simulink library "ddm"  (R2021b)
settings: Solver=VariableStepAuto  StartTime=0.0  StopTime=10.0  RelTol=1e-3
undefined symbols (not defined in the file or in its folder): ADDM_FrTMTqDev_X_Nm, ADDM_RrTMTqDev_X_Nm, ENUM_ADASACCSTA_ERROR, ENUM_ADASACCSTA_OFF, ENUM_ADASACCSTA_STANDBY, ENUM_ALLOWMOV_ALLOWREADY, ENUM_APS, ENUM_BRKSTA_ERROR, ENUM_BRKSTA_OFF, ENUM_BRKSTA_ON, ENUM_BRKSW_INVALID, ENUM_BRKSW_OFF, ENUM_BRKSW_ON, ENUM_CHGPREACTERRSTA_OBCPRE, ENUM_DCDCFAULTSTA_ANYFAULTLV1, ENUM_DCDCFAULTSTA_ANYFAULTLV2, ENUM_DRIVETRAIN_AWD, ENUM_DRIVETRAIN_FWD, ENUM_DRIVETRAIN_RWD, ENUM_EDUDRTSTA_NORMAL, ENUM_EPBSTA_APPLIED, ENUM_EPBSTA_RELEASED, ENUM_GEARACTUALPOSN_INVALID, ENUM_GEARACTUALPOSN_P, ENUM_HVBATTREADYPRE_READY, ENUM_MCUWARN_LV0, ENUM_MCUWARN_LV1, ENUM_MCUWARN_LV2, ENUM_MCUWARN_LV3, ENUM_MCUWARN_NOERROR, ENUM_OBCFAULTSTA_ANYFAULT, ENUM_PAS_R2F2, ENUM_PDFAULT_BATTPDFAIL, ENUM_PDFAULT_DCDCDISABLE, ENUM_PDFAULT_MCUDISABLE, ENUM_PDFAULT_MCUDISCHRG, ENUM_POWERSTA_OFF, ENUM_POWERSTA_ON, ENUM_POWERSTA_READY, ENUM_POWERSTA_STANDBY, ENUM_PRESSINDI_LOW, ENUM_PUFAULT_BATTUPFAIL, ENUM_PUFAULT_DCDCENABLEFAIL, ENUM_PUFAULT_PRECHRGCHKFAIL, ENUM_PUFAULT_SAFETYCHKFAIL, ENUM_PUSTATE_COMPLETED, ENUM_PWRSTASW_OFF, ENUM_PWRSTASW_OFFA, ENUM_PWRSTASW_OFFCHVCHRG, ENUM_PWRSTASW_OFFCLVCHRG, ENUM_PWRSTASW_ON, ENUM_PWRSTASW_ONHVCHRG, ENUM_PWRSTASW_READY, ENUM_PWRSTASW_STANDBY, ENUM_SHIFTCOMMAND_P, ENUM_SHIFTERERRSTA_PBUTTONFAILURE, ENUM_VEHMALFUNLV_2ND, ENUM_VEHMALFUNLV_3RD, ENUM_VEHMALFUNLV_4TH, ENUM_VEHMALFUNLV_NORMAL ... (+459)
libraries: hcu_lib x515, simulink x3
(part 10 of 25)

== system ddm/DDM/DDM/TPM/LFWheelTmpHigh ==
  note: Test Detection Criteria
  note: Test Pass Criteria
  note: Release Condition After Decision
  note: Diagnostics and Fault Handling
  task_time_s : Inport
  VPMM_PowerSta_enum : Inport  Port=2
  DTC_clear_request : Inport  Port=3
  VTPM_LFWheelTmpHigh_flg : Inport  Port=4
  Constant : Constant  Value=KDDM_LFWheelTmpHighDTC_cnt
  Constant1 : Constant  Value=KDDM_LFWheelTmpHighDTC_cnt
  Constant10 : Constant  Value=ENUM_POWERSTA_OFF
  Constant11 : Constant  Value=KDDM_LFWheelTmpHighPassSW_flg
  Constant12 : Constant  Value=FALSE
  Constant13 : Constant  Value=KDDM_LFWheelTmpHighCFSSW_flg
  Constant14 : Constant  Value=KDDM_LFWheelTmpHighDFSSW_flg
  Constant15 : Constant  Value=KDDM_LFWheelTmpHighPassTO_s
  Constant2 : Constant  Value=ENUM_POWERSTA_READY
  Constant24 : Constant  Value=TRUE
  Constant25 : Constant  Value=FALSE
  Constant3 : Constant  Value=ENUM_POWERSTA_ON
  Constant4 : Constant  Value=FALSE
  Constant46 : Constant  Value=KDDM_LFWheelTmpHighDetSW_flg
  Constant5 : Constant  Value=ENUM_POWERSTA_READY
  Constant6 : Constant  Value=KDDM_LFWheelTmpHighDetTO_s
  Constant7 : Constant  Value=ENUM_POWERSTA_ON
  Constant8 : Constant  Value=TRUE
  Constant9 : Constant  Value=KDDM_LFWheelTmpHighPassTO_s
  DTC_Couter : hcu_lib/Basic_Blocks/DTC_Couter
  DTC_Info : hcu_lib/Basic_Blocks/DTC_Info
  Data Type Conversion1 : DataTypeConversion  OutDataTypeStr=uint8
  Equal{1..5} (5 alike) : RelationalOperator  Operator===  OutDataTypeStr=boolean  RndMeth=Simplest
  Equal6 : RelationalOperator  OutDataTypeStr=boolean  RndMeth=Simplest
  Logical Operator{1,4..5,7..8} (5 alike) : Logic  Operator=OR  AllPortsSameDT=off  OutDataTypeStr=boolean
  Logical Operator12 : Logic  AllPortsSameDT=off  OutDataTypeStr=boolean
  Logical Operator15 : Logic  AllPortsSameDT=off  OutDataTypeStr=boolean
  Logical Operator18 : Logic  AllPortsSameDT=off  OutDataTypeStr=boolean
  Logical Operator19 : Logic  Inputs=3  AllPortsSameDT=off  OutDataTypeStr=boolean
  Logical Operator2 : Logic  Operator=NOT  AllPortsSameDT=off  OutDataTypeStr=boolean
  Logical Operator3 : Logic  Operator=OR  Inputs=3  AllPortsSameDT=off  OutDataTypeStr=boolean
  Logical Operator6 : Logic  Operator=NOT  AllPortsSameDT=off  OutDataTypeStr=boolean
  Relay : Relay  OnSwitchValue=ONE_INT  OffSwitchValue=ZERO_INT
  SR_Latch1 : Subsystem  mask(SR_Latch){}
      mask help: SR latch function.
  SR_Latch3 : hcu_lib/Basic_Blocks/SR_Latch
  SR_Latch4 : hcu_lib/Basic_Blocks/SR_Latch
  Switch{2..4,6} (4 alike) : Switch  Criteria=u2 ~= 0
  Test Detection Criteria : hcu_lib/Basic_Blocks/Test Detection Criteria
  Timer1 : hcu_lib/Basic_Blocks/Timer
  VDDM_LFWheelTmpHighDTC_raw32 : Outport
  wires:
  [VTPM_LFWheelTmpHigh_flg] -> Switch4/1
  [VTPM_LFWheelTmpHigh_flg] -> Switch3/1
  task_time_s/1 -> [task_time_s]
  VPMM_PowerSta_enum/1 -> [VPMM_PowerSta_enum]
  Logical Operator8/1 -> Switch2/2
  Constant25/1 -> Switch2/3
  Switch2/1 -> [VDDM_LFWheelTmpHighCFSRls_flg]
  [DTC_clear_request] -> Logical Operator8/2
  Constant24/1 -> Switch2/1
  Constant10/1 -> Equal4/2
  Equal4/1 -> Logical Operator8/1
  [VDDM_LFWheelTmpHighDTC_cnt] -> Relay/1
  [VDDM_LFWheelTmpHighCFS_flg] -> Logical Operator7/1
  Logical Operator3/1 -> Logical Operator15/1
  [VDDM_LFWheelTmpHighDet_flg] -> Logical Operator19/1
  Relay/1 -> SR_Latch3/1
  DTC_Couter/2 -> Data Type Conversion1/1
  Constant1/1 -> DTC_Couter/3
  Logical Operator15/1 -> DTC_Couter/2
  Constant11/1 -> Logical Operator15/2
  Logical Operator19/1 -> DTC_Couter/1
  Constant46/1 -> Logical Operator19/2
  Data Type Conversion1/1 -> [VDDM_LFWheelTmpHighDTC_cnt]  "VDDM_LFWheelTmpHighDTC_cnt"
  DTC_Couter/1 -> SR_Latch4/1
  [VDDM_LFWheelTmpHighPass_flg] -> Logical Operator3/2
  [VDDM_LFWheelTmpHighCFSRls_flg] -> Logical Operator5/1
  SR_Latch4/1 -> Logical Operator18/1
  Logical Operator12/1 -> [VDDM_LFWheelTmpHighDFS_flg]
  Constant13/1 -> Logical Operator18/2
  SR_Latch3/1 -> Logical Operator12/2
  Constant14/1 -> Logical Operator12/1
  Logical Operator18/1 -> [VDDM_LFWheelTmpHighCFS_flg]
  [VDDM_LFWheelTmpHighCFSRls_flg] -> Logical Operator3/3
  DTC_clear_request/1 -> [DTC_clear_request]
  [VPMM_PowerSta_enum] -> Equal4/1
  [VDDM_LFWheelTmpHighCFS_flg] -> DTC_Info/3
  DTC_Info/1 -> VDDM_LFWheelTmpHighDTC_raw32/1  "VDDM_LFWheelTmpHighDTC_raw32"
  Test Detection Criteria/1 -> [VDDM_LFWheelTmpHighDet_flg]  "VDDM_LFWheelTmpHighDet_flg"
  [VDDM_LFWheelTmpHighDet_flg] -> DTC_Info/1
  [VDDM_LFWheelTmpHighPass_flg] -> DTC_Info/2
  [DTC_clear_request] -> DTC_Info/4
  [VPMM_PowerSta_enum] -> Equal1/1
  Constant4/1 -> Switch3/3
  Constant5/1 -> Equal1/2
  Constant7/1 -> Equal5/2
  Logical Operator1/1 -> Switch3/2
  Equal5/1 -> Logical Operator1/1
  Equal1/1 -> Logical Operator1/2
  [VPMM_PowerSta_enum] -> Equal5/1
  Constant6/1 -> Test Detection Criteria/4
  Constant/1 -> Test Detection Criteria/3
  [task_time_s] -> Test Detection Criteria/2
  [VPMM_PowerSta_enum] -> Equal3/1
  Equal2/1 -> Logical Operator4/2
  Constant8/1 -> Switch4/3
  Constant2/1 -> Equal2/2
  Constant3/1 -> Equal3/2
  [VPMM_PowerSta_enum] -> Equal2/1
  Equal3/1 -> Logical Operator4/1
  Logical Operator4/1 -> Switch4/2
  VTPM_LFWheelTmpHigh_flg/1 -> [VTPM_LFWheelTmpHigh_flg]
  Switch3/1 -> [VDDM_LFWheelTmpHighChk_flg], Switch6/3
  [DTC_clear_request] -> Switch6/2
  Constant12/1 -> Switch6/1
  Switch6/1 -> Test Detection Criteria/1
  Switch4/1 -> Timer1/2, Logical Operator6/1
  Equal6/1 -> SR_Latch1/1(set)
  Constant9/1 -> Equal6/2
  SR_Latch1/1(latched) -> [VDDM_LFWheelTmpHighPass_flg]
  [VDDM_LFWheelTmpHighChk_flg] -> SR_Latch1/2(reset)
  [task_time_s] -> Timer1/3
  Timer1/1 -> Equal6/1
  Constant15/1 -> Timer1/4
  Logical Operator6/1 -> Timer1/1
  Logical Operator2/1 -> Logical Operator19/3
  [DTC_clear_request] -> Logical Operator3/1, Logical Operator2/1
  Logical Operator5/1 -> SR_Latch4/2
  [DTC_clear_request] -> Logical Operator5/2
  Logical Operator7/1 -> SR_Latch3/2
  [DTC_clear_request] -> Logical Operator7/2

== system ddm/DDM/DDM/TPM/LRBatwarn ==
  note: Test Detection Criteria
  note: Test Pass Criteria
  note: Release Condition After Decision
  note: Diagnostics and Fault Handling
  task_time_s : Inport
  VPMM_PowerSta_enum : Inport  Port=2
  DTC_clear_request : Inport  Port=3
  VTPM_LRBatwarn_flg : Inport  Port=4
  Constant : Constant  Value=KDDM_LRBatwarnDTC_cnt
  Constant1 : Constant  Value=KDDM_LRBatwarnDTC_cnt
  Constant10 : Constant  Value=ENUM_POWERSTA_OFF
  Constant11 : Constant  Value=KDDM_LRBatwarnPassSW_flg
  Constant12 : Constant  Value=FALSE
  Constant13 : Constant  Value=KDDM_LRBatwarnCFSSW_flg
  Constant14 : Constant  Value=KDDM_LRBatwarnDFSSW_flg
  Constant15 : Constant  Value=KDDM_LRBatwarnPassTO_s
  Constant2 : Constant  Value=ENUM_POWERSTA_READY
  Constant24 : Constant  Value=TRUE
  Constant25 : Constant  Value=FALSE
  Constant3 : Constant  Value=ENUM_POWERSTA_ON
  Constant4 : Constant  Value=FALSE
  Constant46 : Constant  Value=KDDM_LRBatwarnDetSW_flg
  Constant5 : Constant  Value=ENUM_POWERSTA_READY
  Constant6 : Constant  Value=KDDM_LRBatwarnDetTO_s
  Constant7 : Constant  Value=ENUM_POWERSTA_ON
  Constant8 : Constant  Value=TRUE
  Constant9 : Constant  Value=KDDM_LRBatwarnPassTO_s
  DTC_Couter : hcu_lib/Basic_Blocks/DTC_Couter
  DTC_Info : hcu_lib/Basic_Blocks/DTC_Info
  Data Type Conversion1 : DataTypeConversion  OutDataTypeStr=uint8
  Equal{1..5} (5 alike) : RelationalOperator  Operator===  OutDataTypeStr=boolean  RndMeth=Simplest
  Equal6 : RelationalOperator  OutDataTypeStr=boolean  RndMeth=Simplest
  Logical Operator{1..2,4,7..8} (5 alike) : Logic  Operator=OR  AllPortsSameDT=off  OutDataTypeStr=boolean
  Logical Operator12 : Logic  AllPortsSameDT=off  OutDataTypeStr=boolean
  Logical Operator15 : Logic  AllPortsSameDT=off  OutDataTypeStr=boolean
  Logical Operator18 : Logic  AllPortsSameDT=off  OutDataTypeStr=boolean
  Logical Operator19 : Logic  Inputs=3  AllPortsSameDT=off  OutDataTypeStr=boolean
  Logical Operator3 : Logic  Operator=OR  Inputs=3  AllPortsSameDT=off  OutDataTypeStr=boolean
  Logical Operator5 : Logic  Operator=NOT  AllPortsSameDT=off  OutDataTypeStr=boolean
  Logical Operator6 : Logic  Operator=NOT  AllPortsSameDT=off  OutDataTypeStr=boolean
  Relay : Relay  OnSwitchValue=ONE_INT  OffSwitchValue=ZERO_INT
  SR_Latch1 : Subsystem  mask(SR_Latch){}
      mask help: SR latch function.
  SR_Latch3 : hcu_lib/Basic_Blocks/SR_Latch
  SR_Latch4 : hcu_lib/Basic_Blocks/SR_Latch
  Switch{2..4,6} (4 alike) : Switch  Criteria=u2 ~= 0
  Test Detection Criteria : hcu_lib/Basic_Blocks/Test Detection Criteria
  Timer1 : hcu_lib/Basic_Blocks/Timer
  VDDM_LRBatwarnDTC_raw32 : Outport
  wires:
  task_time_s/1 -> [task_time_s]
  VPMM_PowerSta_enum/1 -> [VPMM_PowerSta_enum]
  Logical Operator8/1 -> Switch2/2
  Constant25/1 -> Switch2/3
  Switch2/1 -> [VDDM_LRBatwarnCFSRls_flg]
  [DTC_clear_request] -> Logical Operator8/2
  Constant24/1 -> Switch2/1
  Constant10/1 -> Equal4/2
  Equal4/1 -> Logical Operator8/1
  [VDDM_LRBatwarnDTC_cnt] -> Relay/1
  [VDDM_LRBatwarnCFS_flg] -> Logical Operator7/1
  Logical Operator3/1 -> Logical Operator15/1
  [VDDM_LRBatwarnDet_flg] -> Logical Operator19/1
  Relay/1 -> SR_Latch3/1
  DTC_Couter/2 -> Data Type Conversion1/1
  Constant1/1 -> DTC_Couter/3
  Logical Operator15/1 -> DTC_Couter/2
  Constant11/1 -> Logical Operator15/2
  Logical Operator19/1 -> DTC_Couter/1
  Constant46/1 -> Logical Operator19/2
  Data Type Conversion1/1 -> [VDDM_LRBatwarnDTC_cnt]  "VDDM_LRBatwarnDTC_cnt"
  DTC_Couter/1 -> SR_Latch4/1
  [VDDM_LRBatwarnPass_flg] -> Logical Operator3/2
  [VDDM_LRBatwarnCFSRls_flg] -> Logical Operator2/1
  SR_Latch4/1 -> Logical Operator18/1
  Logical Operator12/1 -> [VDDM_LRBatwarnDFS_flg]
  Constant13/1 -> Logical Operator18/2
  SR_Latch3/1 -> Logical Operator12/2
  Constant14/1 -> Logical Operator12/1
  Logical Operator18/1 -> [VDDM_LRBatwarnCFS_flg]
  [VDDM_LRBatwarnCFSRls_flg] -> Logical Operator3/3
  DTC_clear_request/1 -> [DTC_clear_request]
  [VPMM_PowerSta_enum] -> Equal4/1
  [VDDM_LRBatwarnCFS_flg] -> DTC_Info/3
  DTC_Info/1 -> VDDM_LRBatwarnDTC_raw32/1  "VDDM_LRBatwarnDTC_raw32"
  Test Detection Criteria/1 -> [VDDM_LRBatwarnDet_flg]  "VDDM_LRBatwarnDet_flg"
  [VDDM_LRBatwarnDet_flg] -> DTC_Info/1
  [VDDM_LRBatwarnPass_flg] -> DTC_Info/2
  [DTC_clear_request] -> DTC_Info/4
  [VPMM_PowerSta_enum] -> Equal1/1
  Constant4/1 -> Switch3/3
  Constant2/1 -> Equal1/2
  Constant3/1 -> Equal5/2
  Logical Operator1/1 -> Switch3/2
  Equal5/1 -> Logical Operator1/1
  Equal1/1 -> Logical Operator1/2
  [VPMM_PowerSta_enum] -> Equal5/1
  Constant6/1 -> Test Detection Criteria/4
  Constant/1 -> Test Detection Criteria/3
  [task_time_s] -> Test Detection Criteria/2
  [VTPM_LRBatwarn_flg] -> Switch3/1
  [VPMM_PowerSta_enum] -> Equal3/1
  Equal2/1 -> Logical Operator4/2
  Constant8/1 -> Switch4/3
  Constant5/1 -> Equal2/2
  Constant7/1 -> Equal3/2
  [VPMM_PowerSta_enum] -> Equal2/1
  Equal3/1 -> Logical Operator4/1
  Logical Operator4/1 -> Switch4/2
  [VTPM_LRBatwarn_flg] -> Switch4/1
  VTPM_LRBatwarn_flg/1 -> [VTPM_LRBatwarn_flg]
  [DTC_clear_request] -> Switch6/2
  Constant12/1 -> Switch6/1
  Switch6/1 -> Test Detection Criteria/1
  Switch4/1 -> Timer1/2, Logical Operator6/1
  Equal6/1 -> SR_Latch1/1(set)
  [VDDM_LRBatwarnChk_flg] -> SR_Latch1/2(reset)
  Timer1/1 -> Equal6/1
  Constant9/1 -> Equal6/2
  SR_Latch1/1(latched) -> [VDDM_LRBatwarnPass_flg]
  [task_time_s] -> Timer1/3
  Logical Operator6/1 -> Timer1/1
  Constant15/1 -> Timer1/4
  Switch3/1 -> [VDDM_LRBatwarnChk_flg], Switch6/3
  Logical Operator5/1 -> Logical Operator19/3
  [DTC_clear_request] -> Logical Operator3/1, Logical Operator5/1
  Logical Operator2/1 -> SR_Latch4/2
  [DTC_clear_request] -> Logical Operator2/2
  Logical Operator7/1 -> SR_Latch3/2
  [DTC_clear_request] -> Logical Operator7/2

== system ddm/DDM/DDM/TPM/LRPressureLow ==
  note: Diagnostics and Fault Handling
  note: Release Condition After Decision
  note: Test Pass Criteria
  note: Test Detection Criteria
  task_time_s : Inport
  VPMM_PowerSta_enum : Inport  Port=2
  DTC_clear_request : Inport  Port=3
  VTPM_LRPressIndi_enum : Inport  Port=4
  Constant : Constant  Value=KDDM_LRPressIndiDTC_cnt
  Constant1 : Constant  Value=KDDM_LRPressIndiDTC_cnt
  Constant10 : Constant  Value=ENUM_POWERSTA_OFF
  Constant11 : Constant  Value=KDDM_LRPressIndiPassSW_flg
  Constant12 : Constant  Value=FALSE
  Constant13 : Constant  Value=KDDM_LRPressIndiCFSSW_flg
  Constant14 : Constant  Value=KDDM_LRPressIndiDFSSW_flg
  Constant15 : Constant  Value=KDDM_LRPressIndiPassTO_s
  Constant16 : Constant  Value=ENUM_PRESSINDI_LOW
  Constant17 : Constant  Value=ENUM_PRESSINDI_LOW
  Constant2 : Constant  Value=ENUM_POWERSTA_READY
  Constant24 : Constant  Value=TRUE
  Constant25 : Constant  Value=FALSE
  Constant3 : Constant  Value=ENUM_POWERSTA_ON
  Constant4 : Constant  Value=FALSE
  Constant46 : Constant  Value=KDDM_LRPressIndiDetSW_flg
  Constant5 : Constant  Value=ENUM_POWERSTA_READY
  Constant6 : Constant  Value=KDDM_LRPressIndiDetTO_s
  Constant7 : Constant  Value=ENUM_POWERSTA_ON
  Constant8 : Constant  Value=TRUE
  Constant9 : Constant  Value=KDDM_LRPressIndiPassTO_s
  DTC_Couter : hcu_lib/Basic_Blocks/DTC_Couter
  DTC_Info : hcu_lib/Basic_Blocks/DTC_Info
  Data Type Conversion1 : DataTypeConversion  OutDataTypeStr=uint8
  Equal{1..5,7..8} (7 alike) : RelationalOperator  Operator===  OutDataTypeStr=boolean  RndMeth=Simplest
  Equal6 : RelationalOperator  OutDataTypeStr=boolean  RndMeth=Simplest
  Logical Operator{1,4..5,7..8} (5 alike) : Logic  Operator=OR  AllPortsSameDT=off  OutDataTypeStr=boolean
  Logical Operator12 : Logic  AllPortsSameDT=off  OutDataTypeStr=boolean
  Logical Operator15 : Logic  AllPortsSameDT=off  OutDataTypeStr=boolean
  Logical Operator18 : Logic  AllPortsSameDT=off  OutDataTypeStr=boolean
  Logical Operator19 : Logic  Inputs=3  AllPortsSameDT=off  OutDataTypeStr=boolean
  Logical Operator2 : Logic  Operator=NOT  AllPortsSameDT=off  OutDataTypeStr=boolean
  Logical Operator3 : Logic  Operator=OR  Inputs=3  AllPortsSameDT=off  OutDataTypeStr=boolean
  Logical Operator6 : Logic  Operator=NOT  AllPortsSameDT=off  OutDataTypeStr=boolean
  Relay : Relay  OnSwitchValue=ONE_INT  OffSwitchValue=ZERO_INT
  SR_Latch1 : Subsystem  mask(SR_Latch){}
      mask help: SR latch function.
  SR_Latch3 : hcu_lib/Basic_Blocks/SR_Latch
  SR_Latch4 : hcu_lib/Basic_Blocks/SR_Latch
  Switch{2..4,6} (4 alike) : Switch  Criteria=u2 ~= 0
  Test Detection Criteria : hcu_lib/Basic_Blocks/Test Detection Criteria
  Timer1 : hcu_lib/Basic_Blocks/Timer
  VDDM_LRPressIndiDTC_raw32 : Outport
  wires:
  Logical Operator6/1 -> Timer1/1
  Constant15/1 -> Timer1/4
  Timer1/1 -> Equal6/1
  [task_time_s] -> Timer1/3
  [VDDM_LRPressIndiChk_flg] -> SR_Latch1/2(reset)
  SR_Latch1/1(latched) -> [VDDM_LRPressIndiPass_flg]
  Constant9/1 -> Equal6/2
  Equal6/1 -> SR_Latch1/1(set)
  Switch4/1 -> Timer1/2, Logical Operator6/1
  Switch6/1 -> Test Detection Criteria/1
  Constant12/1 -> Switch6/1
  [DTC_clear_request] -> Switch6/2
  Switch3/1 -> Switch6/3, [VDDM_LRPressIndiChk_flg]
  VTPM_LRPressIndi_enum/1 -> [VTPM_LRPressIndi_enum]
  Logical Operator4/1 -> Switch4/2
  Equal3/1 -> Logical Operator4/1
  [VPMM_PowerSta_enum] -> Equal2/1
  Constant3/1 -> Equal3/2
  Constant2/1 -> Equal2/2
  Constant8/1 -> Switch4/3
  Equal2/1 -> Logical Operator4/2
  [VPMM_PowerSta_enum] -> Equal3/1
  [task_time_s] -> Test Detection Criteria/2
  Constant/1 -> Test Detection Criteria/3
  Constant6/1 -> Test Detection Criteria/4
  [VPMM_PowerSta_enum] -> Equal5/1
  Equal1/1 -> Logical Operator1/2
  Equal5/1 -> Logical Operator1/1
  Logical Operator1/1 -> Switch3/2
  Constant7/1 -> Equal5/2
  Constant5/1 -> Equal1/2
  Constant4/1 -> Switch3/3
  [VPMM_PowerSta_enum] -> Equal1/1
  [DTC_clear_request] -> DTC_Info/4
  [VDDM_LRPressIndiPass_flg] -> DTC_Info/2
  [VDDM_LRPressIndiDet_flg] -> DTC_Info/1
  Test Detection Criteria/1 -> [VDDM_LRPressIndiDet_flg]  "VDDM_LRPressIndiDet_flg"
  DTC_Info/1 -> VDDM_LRPressIndiDTC_raw32/1  "VDDM_LRPressIndiDTC_raw32"
  [VDDM_LRPressIndiCFS_flg] -> DTC_Info/3
  [VPMM_PowerSta_enum] -> Equal4/1
  DTC_clear_request/1 -> [DTC_clear_request]
  [VDDM_LRPressIndiCFSRls_flg] -> Logical Operator3/3
  Logical Operator18/1 -> [VDDM_LRPressIndiCFS_flg]
  Constant14/1 -> Logical Operator12/1
  SR_Latch3/1 -> Logical Operator12/2
  Constant13/1 -> Logical Operator18/2
  Logical Operator12/1 -> [VDDM_LRPressIndiDFS_flg]
  SR_Latch4/1 -> Logical Operator18/1
  [VDDM_LRPressIndiCFSRls_flg] -> Logical Operator5/1
  [VDDM_LRPressIndiPass_flg] -> Logical Operator3/2
  DTC_Couter/1 -> SR_Latch4/1
  Data Type Conversion1/1 -> [VDDM_LRPressIndiDTC_cnt]  "VDDM_LRPressIndiDTC_cnt"
  Constant46/1 -> Logical Operator19/2
  Logical Operator19/1 -> DTC_Couter/1
  Constant11/1 -> Logical Operator15/2
  Logical Operator15/1 -> DTC_Couter/2
  Constant1/1 -> DTC_Couter/3
  DTC_Couter/2 -> Data Type Conversion1/1
  Relay/1 -> SR_Latch3/1
  [VDDM_LRPressIndiDet_flg] -> Logical Operator19/1
  Logical Operator3/1 -> Logical Operator15/1
  [VDDM_LRPressIndiCFS_flg] -> Logical Operator7/1
  [VDDM_LRPressIndiDTC_cnt] -> Relay/1
  Equal4/1 -> Logical Operator8/1
  Constant10/1 -> Equal4/2
  Constant24/1 -> Switch2/1
  [DTC_clear_request] -> Logical Operator8/2
  Switch2/1 -> [VDDM_LRPressIndiCFSRls_flg]
  Constant25/1 -> Switch2/3
  Logical Operator8/1 -> Switch2/2
  VPMM_PowerSta_enum/1 -> [VPMM_PowerSta_enum]
  task_time_s/1 -> [task_time_s]
  [VTPM_LRPressIndi_enum] -> Equal7/1
  Equal7/1 -> Switch3/1
  Constant16/1 -> Equal7/2
  Equal8/1 -> Switch4/1
  Constant17/1 -> Equal8/2
  [VTPM_LRPressIndi_enum] -> Equal8/1
  Logical Operator2/1 -> Logical Operator19/3
  [DTC_clear_request] -> Logical Operator3/1, Logical Operator2/1
  Logical Operator5/1 -> SR_Latch4/2
  [DTC_clear_request] -> Logical Operator5/2
  Logical Operator7/1 -> SR_Latch3/2
  [DTC_clear_request] -> Logical Operator7/2

== system ddm/DDM/DDM/TPM/LRSensorfail ==
  note: Diagnostics and Fault Handling
  note: Release Condition After Decision
  note: Test Pass Criteria
  note: Test Detection Criteria
  task_time_s : Inport
  VPMM_PowerSta_enum : Inport  Port=2
  DTC_clear_request : Inport  Port=3
  VTPM_LRSensorFail_flg : Inport  Port=4
  Constant : Constant  Value=KDDM_LRSensorFailDTC_cnt
  Constant1 : Constant  Value=KDDM_LRSensorFailDTC_cnt
  Constant10 : Constant  Value=ENUM_POWERSTA_OFF
  Constant11 : Constant  Value=KDDM_LRSensorFailPassSW_flg
  Constant12 : Constant  Value=FALSE
  Constant13 : Constant  Value=KDDM_LRSensorFailCFSSW_flg
  Constant14 : Constant  Value=KDDM_LRSensorFailDFSSW_flg
  Constant15 : Constant  Value=KDDM_LRSensorFailPassTO_s
  Constant2 : Constant  Value=ENUM_POWERSTA_READY
  Constant24 : Constant  Value=TRUE
  Constant25 : Constant  Value=FALSE
  Constant3 : Constant  Value=ENUM_POWERSTA_ON
  Constant4 : Constant  Value=FALSE
  Constant46 : Constant  Value=KDDM_LRSensorFailDetSW_flg
  Constant5 : Constant  Value=ENUM_POWERSTA_READY
  Constant6 : Constant  Value=KDDM_LRSensorFailDetTO_s
  Constant7 : Constant  Value=ENUM_POWERSTA_ON
  Constant8 : Constant  Value=TRUE
  Constant9 : Constant  Value=KDDM_LRSensorFailPassTO_s
  DTC_Couter : hcu_lib/Basic_Blocks/DTC_Couter
  DTC_Info : hcu_lib/Basic_Blocks/DTC_Info
  Data Type Conversion1 : DataTypeConversion  OutDataTypeStr=uint8
  Equal{1..5} (5 alike) : RelationalOperator  Operator===  OutDataTypeStr=boolean  RndMeth=Simplest
  Equal6 : RelationalOperator  OutDataTypeStr=boolean  RndMeth=Simplest
  Logical Operator{1,4..5,7..8} (5 alike) : Logic  Operator=OR  AllPortsSameDT=off  OutDataTypeStr=boolean
  Logical Operator12 : Logic  AllPortsSameDT=off  OutDataTypeStr=boolean
  Logical Operator15 : Logic  AllPortsSameDT=off  OutDataTypeStr=boolean
  Logical Operator18 : Logic  AllPortsSameDT=off  OutDataTypeStr=boolean
  Logical Operator19 : Logic  Inputs=3  AllPortsSameDT=off  OutDataTypeStr=boolean
  Logical Operator2 : Logic  Operator=NOT  AllPortsSameDT=off  OutDataTypeStr=boolean
  Logical Operator3 : Logic  Operator=OR  Inputs=3  AllPortsSameDT=off  OutDataTypeStr=boolean
  Logical Operator6 : Logic  Operator=NOT  AllPortsSameDT=off  OutDataTypeStr=boolean
  Relay : Relay  OnSwitchValue=ONE_INT  OffSwitchValue=ZERO_INT
  SR_Latch1 : Subsystem  mask(SR_Latch){}
      mask help: SR latch function.
  SR_Latch3 : hcu_lib/Basic_Blocks/SR_Latch
  SR_Latch4 : hcu_lib/Basic_Blocks/SR_Latch
  Switch{2..4,6} (4 alike) : Switch  Criteria=u2 ~= 0
  Test Detection Criteria : hcu_lib/Basic_Blocks/Test Detection Criteria
  Timer1 : hcu_lib/Basic_Blocks/Timer
  VDDM_LRSensorFailDTC_raw32 : Outport
  wires:
  Logical Operator6/1 -> Timer1/1
  Constant15/1 -> Timer1/4
  Timer1/1 -> Equal6/1
  [task_time_s] -> Timer1/3
  [VDDM_LRSensorFailChk_flg] -> SR_Latch1/2(reset)
  SR_Latch1/1(latched) -> [VDDM_LRSensorFailPass_flg]
  Constant9/1 -> Equal6/2
  Equal6/1 -> SR_Latch1/1(set)
  Switch4/1 -> Logical Operator6/1, Timer1/2
  Switch6/1 -> Test Detection Criteria/1
  Constant12/1 -> Switch6/1
  [DTC_clear_request] -> Switch6/2
  Switch3/1 -> Switch6/3, [VDDM_LRSensorFailChk_flg]
  VTPM_LRSensorFail_flg/1 -> [VTPM_LRSensorFail_flg]
  Logical Operator4/1 -> Switch4/2
  Equal3/1 -> Logical Operator4/1
  [VPMM_PowerSta_enum] -> Equal2/1
  Constant3/1 -> Equal3/2
  Constant2/1 -> Equal2/2
  Constant8/1 -> Switch4/3
  Equal2/1 -> Logical Operator4/2
  [VPMM_PowerSta_enum] -> Equal3/1
  [task_time_s] -> Test Detection Criteria/2
  Constant/1 -> Test Detection Criteria/3
  Constant6/1 -> Test Detection Criteria/4
  [VPMM_PowerSta_enum] -> Equal5/1
  Equal1/1 -> Logical Operator1/2
  Equal5/1 -> Logical Operator1/1
  Logical Operator1/1 -> Switch3/2
  Constant7/1 -> Equal5/2
  Constant5/1 -> Equal1/2
  Constant4/1 -> Switch3/3
  [VPMM_PowerSta_enum] -> Equal1/1
  [DTC_clear_request] -> DTC_Info/4
  [VDDM_LRSensorFailPass_flg] -> DTC_Info/2
  [VDDM_LRSensorFailDet_flg] -> DTC_Info/1
  Test Detection Criteria/1 -> [VDDM_LRSensorFailDet_flg]  "VDDM_LRSensorFailDet_flg"
  DTC_Info/1 -> VDDM_LRSensorFailDTC_raw32/1  "VDDM_LRSensorFailDTC_raw32"
  [VDDM_LRSensorFailCFS_flg] -> DTC_Info/3
  [VPMM_PowerSta_enum] -> Equal4/1
  DTC_clear_request/1 -> [DTC_clear_request]
  [VDDM_LRSensorFailCFSRls_flg] -> Logical Operator3/3
  Logical Operator18/1 -> [VDDM_LRSensorFailCFS_flg]
  Constant14/1 -> Logical Operator12/1
  SR_Latch3/1 -> Logical Operator12/2
  Constant13/1 -> Logical Operator18/2
  Logical Operator12/1 -> [VDDM_LRSensorFailDFS_flg]
  SR_Latch4/1 -> Logical Operator18/1
  [VDDM_LRSensorFailCFSRls_flg] -> Logical Operator5/1
  [VDDM_LRSensorFailPass_flg] -> Logical Operator3/2
  DTC_Couter/1 -> SR_Latch4/1
  Data Type Conversion1/1 -> [VDDM_LRSensorFailDTC_cnt]  "VDDM_LRSensorFailDTC_cnt"
  Constant46/1 -> Logical Operator19/2
  Logical Operator19/1 -> DTC_Couter/1
  Constant11/1 -> Logical Operator15/2
  Logical Operator15/1 -> DTC_Couter/2
  Constant1/1 -> DTC_Couter/3
  DTC_Couter/2 -> Data Type Conversion1/1
  Relay/1 -> SR_Latch3/1
  [VDDM_LRSensorFailDet_flg] -> Logical Operator19/1
  Logical Operator3/1 -> Logical Operator15/1
  [VDDM_LRSensorFailCFS_flg] -> Logical Operator7/1
  [VDDM_LRSensorFailDTC_cnt] -> Relay/1
  Equal4/1 -> Logical Operator8/1
  Constant10/1 -> Equal4/2
  Constant24/1 -> Switch2/1
  [DTC_clear_request] -> Logical Operator8/2
  Switch2/1 -> [VDDM_LRSensorFailCFSRls_flg]
  Constant25/1 -> Switch2/3
  Logical Operator8/1 -> Switch2/2
  VPMM_PowerSta_enum/1 -> [VPMM_PowerSta_enum]
  task_time_s/1 -> [task_time_s]
  [VTPM_LRSensorFail_flg] -> Switch3/1
  [VTPM_LRSensorFail_flg] -> Switch4/1
  Logical Operator2/1 -> Logical Operator19/3
  [DTC_clear_request] -> Logical Operator3/1, Logical Operator2/1
  Logical Operator5/1 -> SR_Latch4/2
  [DTC_clear_request] -> Logical Operator5/2
  Logical Operator7/1 -> SR_Latch3/2
  [DTC_clear_request] -> Logical Operator7/2

== system ddm/DDM/DDM/TPM/LRWheelTmpHigh ==
  note: Test Detection Criteria
  note: Test Pass Criteria
  note: Release Condition After Decision
  note: Diagnostics and Fault Handling
  task_time_s : Inport
  VPMM_PowerSta_enum : Inport  Port=2
  DTC_clear_request : Inport  Port=3
  VTPM_LRWheelTmpHigh_flg : Inport  Port=4
  Constant : Constant  Value=KDDM_LRWheelTmpHighDTC_cnt
  Constant1 : Constant  Value=KDDM_LRWheelTmpHighDTC_cnt
  Constant10 : Constant  Value=ENUM_POWERSTA_OFF
  Constant11 : Constant  Value=KDDM_LRWheelTmpHighPassSW_flg
  Constant12 : Constant  Value=FALSE
  Constant13 : Constant  Value=KDDM_LRWheelTmpHighCFSSW_flg
  Constant14 : Constant  Value=KDDM_LRWheelTmpHighDFSSW_flg
  Constant15 : Constant  Value=KDDM_LRWheelTmpHighPassTO_s
  Constant2 : Constant  Value=ENUM_POWERSTA_READY
  Constant24 : Constant  Value=TRUE
  Constant25 : Constant  Value=FALSE
  Constant3 : Constant  Value=ENUM_POWERSTA_ON
  Constant4 : Constant  Value=FALSE
  Constant46 : Constant  Value=KDDM_LRWheelTmpHighDetSW_flg
  Constant5 : Constant  Value=ENUM_POWERSTA_READY
  Constant6 : Constant  Value=KDDM_LRWheelTmpHighDetTO_s
  Constant7 : Constant  Value=ENUM_POWERSTA_ON
  Constant8 : Constant  Value=TRUE
  Constant9 : Constant  Value=KDDM_LRWheelTmpHighPassTO_s
  DTC_Couter : hcu_lib/Basic_Blocks/DTC_Couter
  DTC_Info : hcu_lib/Basic_Blocks/DTC_Info
  Data Type Conversion1 : DataTypeConversion  OutDataTypeStr=uint8
  Equal{1..5} (5 alike) : RelationalOperator  Operator===  OutDataTypeStr=boolean  RndMeth=Simplest
  Equal6 : RelationalOperator  OutDataTypeStr=boolean  RndMeth=Simplest
  Logical Operator{1,4..5,7..8} (5 alike) : Logic  Operator=OR  AllPortsSameDT=off  OutDataTypeStr=boolean
  Logical Operator12 : Logic  AllPortsSameDT=off  OutDataTypeStr=boolean
  Logical Operator15 : Logic  AllPortsSameDT=off  OutDataTypeStr=boolean
  Logical Operator18 : Logic  AllPortsSameDT=off  OutDataTypeStr=boolean
  Logical Operator19 : Logic  Inputs=3  AllPortsSameDT=off  OutDataTypeStr=boolean
  Logical Operator2 : Logic  Operator=NOT  AllPortsSameDT=off  OutDataTypeStr=boolean
  Logical Operator3 : Logic  Operator=OR  Inputs=3  AllPortsSameDT=off  OutDataTypeStr=boolean
  Logical Operator6 : Logic  Operator=NOT  AllPortsSameDT=off  OutDataTypeStr=boolean
  Relay : Relay  OnSwitchValue=ONE_INT  OffSwitchValue=ZERO_INT
  SR_Latch1 : Subsystem  mask(SR_Latch){}
      mask help: SR latch function.
  SR_Latch3 : hcu_lib/Basic_Blocks/SR_Latch
  SR_Latch4 : hcu_lib/Basic_Blocks/SR_Latch
  Switch{2..4,6} (4 alike) : Switch  Criteria=u2 ~= 0
  Test Detection Criteria : hcu_lib/Basic_Blocks/Test Detection Criteria
  Timer1 : hcu_lib/Basic_Blocks/Timer
  VDDM_LRWheelTmpHighDTC_raw32 : Outport
  wires:
  [VTPM_LRWheelTmpHigh_flg] -> Switch4/1
  [VTPM_LRWheelTmpHigh_flg] -> Switch3/1
  task_time_s/1 -> [task_time_s]
  VPMM_PowerSta_enum/1 -> [VPMM_PowerSta_enum]
  Logical Operator8/1 -> Switch2/2
  Constant25/1 -> Switch2/3
  Switch2/1 -> [VDDM_LRWheelTmpHighCFSRls_flg]
  [DTC_clear_request] -> Logical Operator8/2
  Constant24/1 -> Switch2/1
  Constant10/1 -> Equal4/2
  Equal4/1 -> Logical Operator8/1
  [VDDM_LRWheelTmpHighDTC_cnt] -> Relay/1
  [VDDM_LRWheelTmpHighCFS_flg] -> Logical Operator7/1
  Logical Operator3/1 -> Logical Operator15/1
  [VDDM_LRWheelTmpHighDet_flg] -> Logical Operator19/1
  Relay/1 -> SR_Latch3/1
  DTC_Couter/2 -> Data Type Conversion1/1
  Constant1/1 -> DTC_Couter/3
  Logical Operator15/1 -> DTC_Couter/2
  Constant11/1 -> Logical Operator15/2
  Logical Operator19/1 -> DTC_Couter/1
  Constant46/1 -> Logical Operator19/2
  Data Type Conversion1/1 -> [VDDM_LRWheelTmpHighDTC_cnt]  "VDDM_LRWheelTmpHighDTC_cnt"
  DTC_Couter/1 -> SR_Latch4/1
  [VDDM_LRWheelTmpHighPass_flg] -> Logical Operator3/2
  [VDDM_LRWheelTmpHighCFSRls_flg] -> Logical Operator5/1
  SR_Latch4/1 -> Logical Operator18/1
  Logical Operator12/1 -> [VDDM_LRWheelTmpHighDFS_flg]
  Constant13/1 -> Logical Operator18/2
  SR_Latch3/1 -> Logical Operator12/2
  Constant14/1 -> Logical Operator12/1
  Logical Operator18/1 -> [VDDM_LRWheelTmpHighCFS_flg]
  [VDDM_LRWheelTmpHighCFSRls_flg] -> Logical Operator3/3
  DTC_clear_request/1 -> [DTC_clear_request]
  [VPMM_PowerSta_enum] -> Equal4/1
  [VDDM_LRWheelTmpHighCFS_flg] -> DTC_Info/3
  DTC_Info/1 -> VDDM_LRWheelTmpHighDTC_raw32/1  "VDDM_LRWheelTmpHighDTC_raw32"
  Test Detection Criteria/1 -> [VDDM_LRWheelTmpHighDet_flg]  "VDDM_LRWheelTmpHighDet_flg"
  [VDDM_LRWheelTmpHighDet_flg] -> DTC_Info/1
  [VDDM_LRWheelTmpHighPass_flg] -> DTC_Info/2
  [DTC_clear_request] -> DTC_Info/4
  [VPMM_PowerSta_enum] -> Equal1/1
  Constant4/1 -> Switch3/3
  Constant5/1 -> Equal1/2
  Constant7/1 -> Equal5/2
  Logical Operator1/1 -> Switch3/2
  Equal5/1 -> Logical Operator1/1
  Equal1/1 -> Logical Operator1/2
  [VPMM_PowerSta_enum] -> Equal5/1
  Constant6/1 -> Test Detection Criteria/4
  Constant/1 -> Test Detection Criteria/3
  [task_time_s] -> Test Detection Criteria/2
  [VPMM_PowerSta_enum] -> Equal3/1
  Equal2/1 -> Logical Operator4/2
  Constant8/1 -> Switch4/3
  Constant2/1 -> Equal2/2
  Constant3/1 -> Equal3/2
  [VPMM_PowerSta_enum] -> Equal2/1
  Equal3/1 -> Logical Operator4/1
  Logical Operator4/1 -> Switch4/2
  VTPM_LRWheelTmpHigh_flg/1 -> [VTPM_LRWheelTmpHigh_flg]
  Switch3/1 -> [VDDM_LRWheelTmpHighChk_flg], Switch6/3
  [DTC_clear_request] -> Switch6/2
  Constant12/1 -> Switch6/1
  Switch6/1 -> Test Detection Criteria/1
  Switch4/1 -> Timer1/2, Logical Operator6/1
  Equal6/1 -> SR_Latch1/1(set)
  Constant9/1 -> Equal6/2
  SR_Latch1/1(latched) -> [VDDM_LRWheelTmpHighPass_flg]
  [VDDM_LRWheelTmpHighChk_flg] -> SR_Latch1/2(reset)
  [task_time_s] -> Timer1/3
  Timer1/1 -> Equal6/1
  Constant15/1 -> Timer1/4
  Logical Operator6/1 -> Timer1/1
  Logical Operator2/1 -> Logical Operator19/3
  [DTC_clear_request] -> Logical Operator3/1, Logical Operator2/1
  [DTC_clear_request] -> Logical Operator5/2
  Logical Operator5/1 -> SR_Latch4/2
  Logical Operator7/1 -> SR_Latch3/2
  [DTC_clear_request] -> Logical Operator7/2

== system ddm/DDM/DDM/TPM/RFBatwarn ==
  note: Diagnostics and Fault Handling
  note: Release Condition After Decision
  note: Test Pass Criteria
  note: Test Detection Criteria
  task_time_s : Inport
  VPMM_PowerSta_enum : Inport  Port=2
  DTC_clear_request : Inport  Port=3
  VTPM_RFBatwarn_flg : Inport  Port=4
  Constant : Constant  Value=KDDM_RFBatwarnDTC_cnt
  Constant1 : Constant  Value=KDDM_RFBatwarnDTC_cnt
  Constant10 : Constant  Value=ENUM_POWERSTA_OFF
  Constant11 : Constant  Value=KDDM_RFBatwarnPassSW_flg
  Constant12 : Constant  Value=FALSE
  Constant13 : Constant  Value=KDDM_RFBatwarnCFSSW_flg
  Constant14 : Constant  Value=KDDM_RFBatwarnDFSSW_flg
  Constant15 : Constant  Value=KDDM_RFBatwarnPassTO_s
  Constant2 : Constant  Value=ENUM_POWERSTA_READY
  Constant24 : Constant  Value=TRUE
  Constant25 : Constant  Value=FALSE
  Constant3 : Constant  Value=ENUM_POWERSTA_ON
  Constant4 : Constant  Value=FALSE
  Constant46 : Constant  Value=KDDM_RFBatwarnDetSW_flg
  Constant5 : Constant  Value=ENUM_POWERSTA_READY
  Constant6 : Constant  Value=KDDM_RFBatwarnDetTO_s
  Constant7 : Constant  Value=ENUM_POWERSTA_ON
  Constant8 : Constant  Value=TRUE
  Constant9 : Constant  Value=KDDM_RFBatwarnPassTO_s
  DTC_Couter : hcu_lib/Basic_Blocks/DTC_Couter
  DTC_Info : hcu_lib/Basic_Blocks/DTC_Info
  Data Type Conversion1 : DataTypeConversion  OutDataTypeStr=uint8
  Equal{1..5} (5 alike) : RelationalOperator  Operator===  OutDataTypeStr=boolean  RndMeth=Simplest
  Equal6 : RelationalOperator  OutDataTypeStr=boolean  RndMeth=Simplest
  Logical Operator{1,4..5,7..8} (5 alike) : Logic  Operator=OR  AllPortsSameDT=off  OutDataTypeStr=boolean
  Logical Operator12 : Logic  AllPortsSameDT=off  OutDataTypeStr=boolean
  Logical Operator15 : Logic  AllPortsSameDT=off  OutDataTypeStr=boolean
  Logical Operator18 : Logic  AllPortsSameDT=off  OutDataTypeStr=boolean
  Logical Operator19 : Logic  Inputs=3  AllPortsSameDT=off  OutDataTypeStr=boolean
  Logical Operator2 : Logic  Operator=NOT  AllPortsSameDT=off  OutDataTypeStr=boolean
  Logical Operator3 : Logic  Operator=OR  Inputs=3  AllPortsSameDT=off  OutDataTypeStr=boolean
  Logical Operator6 : Logic  Operator=NOT  AllPortsSameDT=off  OutDataTypeStr=boolean
  Relay : Relay  OnSwitchValue=ONE_INT  OffSwitchValue=ZERO_INT
  SR_Latch1 : Subsystem  mask(SR_Latch){}
      mask help: SR latch function.
  SR_Latch3 : hcu_lib/Basic_Blocks/SR_Latch
  SR_Latch4 : hcu_lib/Basic_Blocks/SR_Latch
  Switch{2..4,6} (4 alike) : Switch  Criteria=u2 ~= 0
  Test Detection Criteria : hcu_lib/Basic_Blocks/Test Detection Criteria
  Timer1 : hcu_lib/Basic_Blocks/Timer
  VDDM_RFBatwarnDTC_raw32 : Outport
  wires:
  Switch6/1 -> Test Detection Criteria/1
  Constant12/1 -> Switch6/1
  [DTC_clear_request] -> Switch6/2
  Switch3/1 -> [VDDM_RFBatwarnChk_flg], Switch6/3
  VTPM_RFBatwarn_flg/1 -> [VTPM_RFBatwarn_flg]
  [VTPM_RFBatwarn_flg] -> Switch4/1
  Logical Operator4/1 -> Switch4/2
  Equal3/1 -> Logical Operator4/1
  [VPMM_PowerSta_enum] -> Equal2/1
  Constant3/1 -> Equal3/2
  Constant2/1 -> Equal2/2
  Constant8/1 -> Switch4/3
  Equal2/1 -> Logical Operator4/2
  [VPMM_PowerSta_enum] -> Equal3/1
  [VTPM_RFBatwarn_flg] -> Switch3/1
  [task_time_s] -> Test Detection Criteria/2
  Constant/1 -> Test Detection Criteria/3
  Constant6/1 -> Test Detection Criteria/4
  [VPMM_PowerSta_enum] -> Equal5/1
  Equal1/1 -> Logical Operator1/2
  Equal5/1 -> Logical Operator1/1
  Logical Operator1/1 -> Switch3/2
  Constant7/1 -> Equal5/2
  Constant5/1 -> Equal1/2
  Constant4/1 -> Switch3/3
  [VPMM_PowerSta_enum] -> Equal1/1
  [DTC_clear_request] -> DTC_Info/4
  [VDDM_RFBatwarnPass_flg] -> DTC_Info/2
  [VDDM_RFBatwarnDet_flg] -> DTC_Info/1
  Test Detection Criteria/1 -> [VDDM_RFBatwarnDet_flg]  "VDDM_RFBatwarnDet_flg"
  DTC_Info/1 -> VDDM_RFBatwarnDTC_raw32/1  "VDDM_RFBatwarnDTC_raw32"
  [VDDM_RFBatwarnCFS_flg] -> DTC_Info/3
  [VPMM_PowerSta_enum] -> Equal4/1
  DTC_clear_request/1 -> [DTC_clear_request]
  [VDDM_RFBatwarnCFSRls_flg] -> Logical Operator3/3
  Logical Operator18/1 -> [VDDM_RFBatwarnCFS_flg]
  Constant14/1 -> Logical Operator12/1
  SR_Latch3/1 -> Logical Operator12/2
  Constant13/1 -> Logical Operator18/2
  Logical Operator12/1 -> [VDDM_RFBatwarnDFS_flg]
  SR_Latch4/1 -> Logical Operator18/1
  [VDDM_RFBatwarnCFSRls_flg] -> Logical Operator5/1
  [VDDM_RFBatwarnPass_flg] -> Logical Operator3/2
  DTC_Couter/1 -> SR_Latch4/1
  Data Type Conversion1/1 -> [VDDM_RFBatwarnDTC_cnt]  "VDDM_RFBatwarnDTC_cnt"
  Constant46/1 -> Logical Operator19/2
  Logical Operator19/1 -> DTC_Couter/1
  Constant11/1 -> Logical Operator15/2
  Logical Operator15/1 -> DTC_Couter/2
  Constant1/1 -> DTC_Couter/3
  DTC_Couter/2 -> Data Type Conversion1/1
  Relay/1 -> SR_Latch3/1
  [VDDM_RFBatwarnDet_flg] -> Logical Operator19/1
  Logical Operator3/1 -> Logical Operator15/1
  [VDDM_RFBatwarnCFS_flg] -> Logical Operator7/1
  [VDDM_RFBatwarnDTC_cnt] -> Relay/1
  Equal4/1 -> Logical Operator8/1
  Constant10/1 -> Equal4/2
  Constant24/1 -> Switch2/1
  [DTC_clear_request] -> Logical Operator8/2
  Switch2/1 -> [VDDM_RFBatwarnCFSRls_flg]
  Constant25/1 -> Switch2/3
  Logical Operator8/1 -> Switch2/2
  VPMM_PowerSta_enum/1 -> [VPMM_PowerSta_enum]
  task_time_s/1 -> [task_time_s]
  Switch4/1 -> Timer1/2, Logical Operator6/1
  Equal6/1 -> SR_Latch1/1(set)
  [VDDM_RFBatwarnChk_flg] -> SR_Latch1/2(reset)
  Timer1/1 -> Equal6/1
  Constant9/1 -> Equal6/2
  SR_Latch1/1(latched) -> [VDDM_RFBatwarnPass_flg]
  [task_time_s] -> Timer1/3
  Logical Operator6/1 -> Timer1/1
  Constant15/1 -> Timer1/4
  Logical Operator2/1 -> Logical Operator19/3
  [DTC_clear_request] -> Logical Operator3/1, Logical Operator2/1
  Logical Operator5/1 -> SR_Latch4/2
  [DTC_clear_request] -> Logical Operator5/2
  Logical Operator7/1 -> SR_Latch3/2
  [DTC_clear_request] -> Logical Operator7/2

== system ddm/DDM/DDM/TPM/RFPressureLow ==
  note: Test Detection Criteria
  note: Test Pass Criteria
  note: Release Condition After Decision
  note: Diagnostics and Fault Handling
  task_time_s : Inport
  VPMM_PowerSta_enum : Inport  Port=2
  DTC_clear_request : Inport  Port=3
  VTPM_RFPressIndi_enum : Inport  Port=4
  Constant : Constant  Value=KDDM_RFPressIndiDTC_cnt
  Constant1 : Constant  Value=KDDM_RFPressIndiDTC_cnt
  Constant10 : Constant  Value=ENUM_POWERSTA_OFF
  Constant11 : Constant  Value=KDDM_RFPressIndiPassSW_flg
  Constant12 : Constant  Value=FALSE
  Constant13 : Constant  Value=KDDM_RFPressIndiCFSSW_flg
  Constant14 : Constant  Value=KDDM_RFPressIndiDFSSW_flg
  Constant15 : Constant  Value=KDDM_RFPressIndiPassTO_s
  Constant16 : Constant  Value=ENUM_PRESSINDI_LOW
  Constant17 : Constant  Value=ENUM_PRESSINDI_LOW
  Constant2 : Constant  Value=ENUM_POWERSTA_READY
  Constant24 : Constant  Value=TRUE
  Constant25 : Constant  Value=FALSE
  Constant3 : Constant  Value=ENUM_POWERSTA_ON
  Constant4 : Constant  Value=FALSE
  Constant46 : Constant  Value=KDDM_RFPressIndiDetSW_flg
  Constant5 : Constant  Value=ENUM_POWERSTA_READY
  Constant6 : Constant  Value=KDDM_RFPressIndiDetTO_s
  Constant7 : Constant  Value=ENUM_POWERSTA_ON
  Constant8 : Constant  Value=TRUE
  Constant9 : Constant  Value=KDDM_RFPressIndiPassTO_s
  DTC_Couter : hcu_lib/Basic_Blocks/DTC_Couter
  DTC_Info : hcu_lib/Basic_Blocks/DTC_Info
  Data Type Conversion1 : DataTypeConversion  OutDataTypeStr=uint8
  Equal{1..5,7..8} (7 alike) : RelationalOperator  Operator===  OutDataTypeStr=boolean  RndMeth=Simplest
  Equal6 : RelationalOperator  OutDataTypeStr=boolean  RndMeth=Simplest
  Logical Operator{1,4..5,7..8} (5 alike) : Logic  Operator=OR  AllPortsSameDT=off  OutDataTypeStr=boolean
  Logical Operator12 : Logic  AllPortsSameDT=off  OutDataTypeStr=boolean
  Logical Operator15 : Logic  AllPortsSameDT=off  OutDataTypeStr=boolean
  Logical Operator18 : Logic  AllPortsSameDT=off  OutDataTypeStr=boolean
  Logical Operator19 : Logic  Inputs=3  AllPortsSameDT=off  OutDataTypeStr=boolean
  Logical Operator2 : Logic  Operator=NOT  AllPortsSameDT=off  OutDataTypeStr=boolean
  Logical Operator3 : Logic  Operator=OR  Inputs=3  AllPortsSameDT=off  OutDataTypeStr=boolean
  Logical Operator6 : Logic  Operator=NOT  AllPortsSameDT=off  OutDataTypeStr=boolean
  Relay : Relay  OnSwitchValue=ONE_INT  OffSwitchValue=ZERO_INT
  SR_Latch1 : Subsystem  mask(SR_Latch){}
      mask help: SR latch function.
  SR_Latch3 : hcu_lib/Basic_Blocks/SR_Latch
  SR_Latch4 : hcu_lib/Basic_Blocks/SR_Latch
  Switch{2..4,6} (4 alike) : Switch  Criteria=u2 ~= 0
  Test Detection Criteria : hcu_lib/Basic_Blocks/Test Detection Criteria
  Timer1 : hcu_lib/Basic_Blocks/Timer
  VDDM_RFPressIndiDTC_raw32 : Outport
  wires:
  [VTPM_RFPressIndi_enum] -> Equal8/1
  Constant17/1 -> Equal8/2
  Equal8/1 -> Switch4/1
  Constant16/1 -> Equal7/2
  Equal7/1 -> Switch3/1
  [VTPM_RFPressIndi_enum] -> Equal7/1
  task_time_s/1 -> [task_time_s]
  VPMM_PowerSta_enum/1 -> [VPMM_PowerSta_enum]
  Logical Operator8/1 -> Switch2/2
  Constant25/1 -> Switch2/3
  Switch2/1 -> [VDDM_RFPressIndiCFSRls_flg]
  [DTC_clear_request] -> Logical Operator8/2
  Constant24/1 -> Switch2/1
  Constant10/1 -> Equal4/2
  Equal4/1 -> Logical Operator8/1
  [VDDM_RFPressIndiDTC_cnt] -> Relay/1
  [VDDM_RFPressIndiCFS_flg] -> Logical Operator7/1
  Logical Operator3/1 -> Logical Operator15/1
  [VDDM_RFPressIndiDet_flg] -> Logical Operator19/1
  Relay/1 -> SR_Latch3/1
  DTC_Couter/2 -> Data Type Conversion1/1
  Constant1/1 -> DTC_Couter/3
  Logical Operator15/1 -> DTC_Couter/2
  Constant11/1 -> Logical Operator15/2
  Logical Operator19/1 -> DTC_Couter/1
  Constant46/1 -> Logical Operator19/2
  Data Type Conversion1/1 -> [VDDM_RFPressIndiDTC_cnt]  "VDDM_RFPressIndiDTC_cnt"
  DTC_Couter/1 -> SR_Latch4/1
  [VDDM_RFPressIndiPass_flg] -> Logical Operator3/2
  [VDDM_RFPressIndiCFSRls_flg] -> Logical Operator5/1
  SR_Latch4/1 -> Logical Operator18/1
  Logical Operator12/1 -> [VDDM_RFPressIndiDFS_flg]
  Constant13/1 -> Logical Operator18/2
  SR_Latch3/1 -> Logical Operator12/2
  Constant14/1 -> Logical Operator12/1
  Logical Operator18/1 -> [VDDM_RFPressIndiCFS_flg]
  [VDDM_RFPressIndiCFSRls_flg] -> Logical Operator3/3
  DTC_clear_request/1 -> [DTC_clear_request]
  [VPMM_PowerSta_enum] -> Equal4/1
  [VDDM_RFPressIndiCFS_flg] -> DTC_Info/3
  DTC_Info/1 -> VDDM_RFPressIndiDTC_raw32/1  "VDDM_RFPressIndiDTC_raw32"
  Test Detection Criteria/1 -> [VDDM_RFPressIndiDet_flg]  "VDDM_RFPressIndiDet_flg"
  [VDDM_RFPressIndiDet_flg] -> DTC_Info/1
  [VDDM_RFPressIndiPass_flg] -> DTC_Info/2
  [DTC_clear_request] -> DTC_Info/4
  [VPMM_PowerSta_enum] -> Equal1/1
  Constant4/1 -> Switch3/3
  Constant5/1 -> Equal1/2
  Constant7/1 -> Equal5/2
  Logical Operator1/1 -> Switch3/2
  Equal5/1 -> Logical Operator1/1
  Equal1/1 -> Logical Operator1/2
  [VPMM_PowerSta_enum] -> Equal5/1
  Constant6/1 -> Test Detection Criteria/4
  Constant/1 -> Test Detection Criteria/3
  [task_time_s] -> Test Detection Criteria/2
  [VPMM_PowerSta_enum] -> Equal3/1
  Equal2/1 -> Logical Operator4/2
  Constant8/1 -> Switch4/3
  Constant2/1 -> Equal2/2
  Constant3/1 -> Equal3/2
  [VPMM_PowerSta_enum] -> Equal2/1
  Equal3/1 -> Logical Operator4/1
  Logical Operator4/1 -> Switch4/2
  VTPM_RFPressIndi_enum/1 -> [VTPM_RFPressIndi_enum]
  Switch3/1 -> [VDDM_RFPressIndiChk_flg], Switch6/3
  [DTC_clear_request] -> Switch6/2
  Constant12/1 -> Switch6/1
  Switch6/1 -> Test Detection Criteria/1
  Switch4/1 -> Logical Operator6/1, Timer1/2
  Equal6/1 -> SR_Latch1/1(set)
  Constant9/1 -> Equal6/2
  SR_Latch1/1(latched) -> [VDDM_RFPressIndiPass_flg]
  [VDDM_RFPressIndiChk_flg] -> SR_Latch1/2(reset)
  [task_time_s] -> Timer1/3
  Timer1/1 -> Equal6/1
  Constant15/1 -> Timer1/4
  Logical Operator6/1 -> Timer1/1
  Logical Operator2/1 -> Logical Operator19/3
  [DTC_clear_request] -> Logical Operator3/1, Logical Operator2/1
  Logical Operator5/1 -> SR_Latch4/2
  [DTC_clear_request] -> Logical Operator5/2
  Logical Operator7/1 -> SR_Latch3/2
  [DTC_clear_request] -> Logical Operator7/2

== system ddm/DDM/DDM/TPM/RFSensorfail ==
  note: Test Detection Criteria
  note: Test Pass Criteria
  note: Release Condition After Decision
  note: Diagnostics and Fault Handling
  task_time_s : Inport
  VPMM_PowerSta_enum : Inport  Port=2
  DTC_clear_request : Inport  Port=3
  VTPM_RFSensorFail_flg : Inport  Port=4
  Constant : Constant  Value=KDDM_RFSensorFailDTC_cnt
  Constant1 : Constant  Value=KDDM_RFSensorFailDTC_cnt
  Constant10 : Constant  Value=ENUM_POWERSTA_OFF
  Constant11 : Constant  Value=KDDM_RFSensorFailPassSW_flg
  Constant12 : Constant  Value=FALSE
  Constant13 : Constant  Value=KDDM_RFSensorFailCFSSW_flg
  Constant14 : Constant  Value=KDDM_RFSensorFailDFSSW_flg
  Constant15 : Constant  Value=KDDM_RFSensorFailPassTO_s
  Constant2 : Constant  Value=ENUM_POWERSTA_READY
  Constant24 : Constant  Value=TRUE
  Constant25 : Constant  Value=FALSE
  Constant3 : Constant  Value=ENUM_POWERSTA_ON
  Constant4 : Constant  Value=FALSE
  Constant46 : Constant  Value=KDDM_RFSensorFailDetSW_flg
  Constant5 : Constant  Value=ENUM_POWERSTA_READY
  Constant6 : Constant  Value=KDDM_RFSensorFailDetTO_s
  Constant7 : Constant  Value=ENUM_POWERSTA_ON
  Constant8 : Constant  Value=TRUE
  Constant9 : Constant  Value=KDDM_RFSensorFailPassTO_s
  DTC_Couter : hcu_lib/Basic_Blocks/DTC_Couter
  DTC_Info : hcu_lib/Basic_Blocks/DTC_Info
  Data Type Conversion1 : DataTypeConversion  OutDataTypeStr=uint8
  Equal{1..5} (5 alike) : RelationalOperator  Operator===  OutDataTypeStr=boolean  RndMeth=Simplest
  Equal6 : RelationalOperator  OutDataTypeStr=boolean  RndMeth=Simplest
  Logical Operator{1,4..5,7..8} (5 alike) : Logic  Operator=OR  AllPortsSameDT=off  OutDataTypeStr=boolean
  Logical Operator12 : Logic  AllPortsSameDT=off  OutDataTypeStr=boolean
  Logical Operator15 : Logic  AllPortsSameDT=off  OutDataTypeStr=boolean
  Logical Operator18 : Logic  AllPortsSameDT=off  OutDataTypeStr=boolean
  Logical Operator19 : Logic  Inputs=3  AllPortsSameDT=off  OutDataTypeStr=boolean
  Logical Operator2 : Logic  Operator=NOT  AllPortsSameDT=off  OutDataTypeStr=boolean
  Logical Operator3 : Logic  Operator=OR  Inputs=3  AllPortsSameDT=off  OutDataTypeStr=boolean
  Logical Operator6 : Logic  Operator=NOT  AllPortsSameDT=off  OutDataTypeStr=boolean
  Relay : Relay  OnSwitchValue=ONE_INT  OffSwitchValue=ZERO_INT
  SR_Latch1 : Subsystem  mask(SR_Latch){}
      mask help: SR latch function.
  SR_Latch3 : hcu_lib/Basic_Blocks/SR_Latch
  SR_Latch4 : hcu_lib/Basic_Blocks/SR_Latch
  Switch{2..4,6} (4 alike) : Switch  Criteria=u2 ~= 0
  Test Detection Criteria : hcu_lib/Basic_Blocks/Test Detection Criteria
  Timer1 : hcu_lib/Basic_Blocks/Timer
  VDDM_RFSensorFailDTC_raw32 : Outport
  wires:
  [VTPM_RFSensorFail_flg] -> Switch4/1
  [VTPM_RFSensorFail_flg] -> Switch3/1
  task_time_s/1 -> [task_time_s]
  VPMM_PowerSta_enum/1 -> [VPMM_PowerSta_enum]
  Logical Operator8/1 -> Switch2/2
  Constant25/1 -> Switch2/3
  Switch2/1 -> [VDDM_RFSensorFailCFSRls_flg]
  [DTC_clear_request] -> Logical Operator8/2
  Constant24/1 -> Switch2/1
  Constant10/1 -> Equal4/2
  Equal4/1 -> Logical Operator8/1
  [VDDM_RFSensorFailDTC_cnt] -> Relay/1
  [VDDM_RFSensorFailCFS_flg] -> Logical Operator7/1
  Logical Operator3/1 -> Logical Operator15/1
  [VDDM_RFSensorFailDet_flg] -> Logical Operator19/1
  Relay/1 -> SR_Latch3/1
  DTC_Couter/2 -> Data Type Conversion1/1
  Constant1/1 -> DTC_Couter/3
  Logical Operator15/1 -> DTC_Couter/2
  Constant11/1 -> Logical Operator15/2
  Logical Operator19/1 -> DTC_Couter/1
  Constant46/1 -> Logical Operator19/2
  Data Type Conversion1/1 -> [VDDM_RFSensorFailDTC_cnt]  "VDDM_RFSensorFailDTC_cnt"
  DTC_Couter/1 -> SR_Latch4/1
  [VDDM_RFSensorFailPass_flg] -> Logical Operator3/2
  [VDDM_RFSensorFailCFSRls_flg] -> Logical Operator5/1
  SR_Latch4/1 -> Logical Operator18/1
  Logical Operator12/1 -> [VDDM_RFSensorFailDFS_flg]
  Constant13/1 -> Logical Operator18/2
  SR_Latch3/1 -> Logical Operator12/2
  Constant14/1 -> Logical Operator12/1
  Logical Operator18/1 -> [VDDM_RFSensorFailCFS_flg]
  [VDDM_RFSensorFailCFSRls_flg] -> Logical Operator3/3
  DTC_clear_request/1 -> [DTC_clear_request]
  [VPMM_PowerSta_enum] -> Equal4/1
  [VDDM_RFSensorFailCFS_flg] -> DTC_Info/3
  DTC_Info/1 -> VDDM_RFSensorFailDTC_raw32/1  "VDDM_RFSensorFailDTC_raw32"
  Test Detection Criteria/1 -> [VDDM_RFSensorFailDet_flg]  "VDDM_RFSensorFailDet_flg"
  [VDDM_RFSensorFailDet_flg] -> DTC_Info/1
  [VDDM_RFSensorFailPass_flg] -> DTC_Info/2
  [DTC_clear_request] -> DTC_Info/4
  [VPMM_PowerSta_enum] -> Equal1/1
  Constant4/1 -> Switch3/3
  Constant5/1 -> Equal1/2
  Constant7/1 -> Equal5/2
  Logical Operator1/1 -> Switch3/2
  Equal5/1 -> Logical Operator1/1
  Equal1/1 -> Logical Operator1/2
  [VPMM_PowerSta_enum] -> Equal5/1
  Constant6/1 -> Test Detection Criteria/4
  Constant/1 -> Test Detection Criteria/3
  [task_time_s] -> Test Detection Criteria/2
  [VPMM_PowerSta_enum] -> Equal3/1
  Equal2/1 -> Logical Operator4/2
  Constant8/1 -> Switch4/3
  Constant2/1 -> Equal2/2
  Constant3/1 -> Equal3/2
  [VPMM_PowerSta_enum] -> Equal2/1
  Equal3/1 -> Logical Operator4/1
  Logical Operator4/1 -> Switch4/2
  VTPM_RFSensorFail_flg/1 -> [VTPM_RFSensorFail_flg]
  Switch3/1 -> [VDDM_RFSensorFailChk_flg], Switch6/3
  [DTC_clear_request] -> Switch6/2
  Constant12/1 -> Switch6/1
  Switch6/1 -> Test Detection Criteria/1
  Switch4/1 -> Timer1/2, Logical Operator6/1
  Equal6/1 -> SR_Latch1/1(set)
  Constant9/1 -> Equal6/2
  SR_Latch1/1(latched) -> [VDDM_RFSensorFailPass_flg]
  [VDDM_RFSensorFailChk_flg] -> SR_Latch1/2(reset)
  [task_time_s] -> Timer1/3
  Timer1/1 -> Equal6/1
  Constant15/1 -> Timer1/4
  Logical Operator6/1 -> Timer1/1
  Logical Operator2/1 -> Logical Operator19/3
  [DTC_clear_request] -> Logical Operator3/1, Logical Operator2/1
  Logical Operator5/1 -> SR_Latch4/2
  [DTC_clear_request] -> Logical Operator5/2
  Logical Operator7/1 -> SR_Latch3/2
  [DTC_clear_request] -> Logical Operator7/2
